simulink model "manual_model_features"  (R2020b)
settings: Solver=VariableStepAuto  StartTime=0.0  StopTime=10.0  RelTol=1e-3
undefined symbols (not defined in the file): sigbuilder_block
libraries: simulink x141
(part 3 of 3)

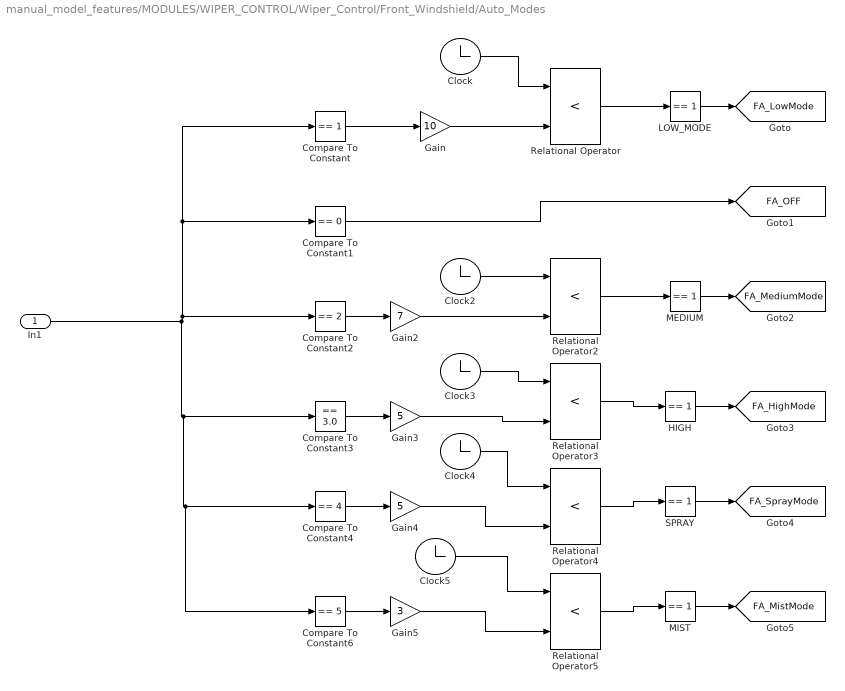
== system manual_model_features/MODULES/WIPER_CONTROL/Wiper_Control/Front_Windshield/Auto_Modes ==
  In1 : Inport
  Clock{,2..5} (5 alike) : Clock
      settings: Decimation=5
  Compare To Constant : simulink/Logic and Bit Operations/Compare To Constant  relop===  const=1  OutDataTypeStr=boolean
  Compare To Constant1 : simulink/Logic and Bit Operations/Compare To Constant  relop===  const=0  OutDataTypeStr=boolean
  Compare To Constant2 : simulink/Logic and Bit Operations/Compare To Constant  relop===  const=2  OutDataTypeStr=boolean
  Compare To Constant3 : simulink/Logic and Bit Operations/Compare To Constant  relop===  const=3.0  OutDataTypeStr=boolean
  Compare To Constant4 : simulink/Logic and Bit Operations/Compare To Constant  relop===  const=4  OutDataTypeStr=boolean
  Compare To Constant6 : simulink/Logic and Bit Operations/Compare To Constant  relop===  const=5  OutDataTypeStr=boolean
  Gain : Gain  Gain=10
  Gain2 : Gain  Gain=7
  Gain3 : Gain  Gain=5
  Gain4 : Gain  Gain=5
  Gain5 : Gain  Gain=3
  HIGH : simulink/Logic and Bit Operations/Compare To Constant  relop===  const=1  OutDataTypeStr=boolean
  LOW_MODE : simulink/Logic and Bit Operations/Compare To Constant  relop===  const=1  OutDataTypeStr=boolean
  MEDIUM : simulink/Logic and Bit Operations/Compare To Constant  relop===  const=1  OutDataTypeStr=boolean
  MIST : simulink/Logic and Bit Operations/Compare To Constant  relop===  const=1  OutDataTypeStr=boolean
  Relational Operator{,2..5} (5 alike) : RelationalOperator  Operator=<  OutDataTypeStr=boolean  RndMeth=Simplest
  SPRAY : simulink/Logic and Bit Operations/Compare To Constant  relop===  const=1  OutDataTypeStr=boolean
  tag scope: FA_HighMode=global, FA_LowMode=global, FA_MediumMode=global, FA_MistMode=global, FA_OFF=global, FA_SprayMode=global
  wires:
  In1/1 -> Compare To Constant6/1, Compare To Constant4/1, Compare To Constant3/1, Compare To Constant2/1, Compare To Constant/1, Compare To Constant1/1
  Clock/1 -> Relational Operator/1
  Relational Operator/1 -> LOW_MODE/1
  Gain/1 -> Relational Operator/2
  Compare To Constant/1 -> Gain/1
  Clock2/1 -> Relational Operator2/1
  Gain2/1 -> Relational Operator2/2
  Compare To Constant2/1 -> Gain2/1
  Clock3/1 -> Relational Operator3/1
  Gain3/1 -> Relational Operator3/2
  Compare To Constant3/1 -> Gain3/1
  Gain4/1 -> Relational Operator4/2
  Clock4/1 -> Relational Operator4/1
  Compare To Constant4/1 -> Gain4/1
  LOW_MODE/1 -> [FA_LowMode]
  MEDIUM/1 -> [FA_MediumMode]
  Relational Operator2/1 -> MEDIUM/1
  HIGH/1 -> [FA_HighMode]
  Relational Operator3/1 -> HIGH/1
  SPRAY/1 -> [FA_SprayMode]
  Relational Operator4/1 -> SPRAY/1
  Compare To Constant1/1 -> [FA_OFF]
  Relational Operator5/1 -> MIST/1
  Gain5/1 -> Relational Operator5/2
  Clock5/1 -> Relational Operator5/1
  MIST/1 -> [FA_MistMode]
  Compare To Constant6/1 -> Gain5/1

== system manual_model_features/MODULES/WIPER_CONTROL/Wiper_Control/Front_Windshield/Manual_mode ==
  In1 : Inport
  Bw30_60 : Logic  IconShape=distinctive  AllPortsSameDT=off  OutDataTypeStr=boolean
  Bw60_100 : Logic  IconShape=distinctive  AllPortsSameDT=off  OutDataTypeStr=boolean
  Compare To Constant1 : simulink/Logic and Bit Operations/Compare To Constant  relop=>  const=30  OutDataTypeStr=boolean
  Compare To Constant2 : simulink/Logic and Bit Operations/Compare To Constant  relop=<=  const=60  OutDataTypeStr=boolean
  Compare To Constant3 : simulink/Logic and Bit Operations/Compare To Constant  relop=>  const=60  OutDataTypeStr=boolean
  Compare To Constant4 : simulink/Logic and Bit Operations/Compare To Constant  relop=<=  const=100  OutDataTypeStr=boolean
  Display : Display
  LessThan30 : simulink/Logic and Bit Operations/Compare To Constant  relop=<=  const=30  OutDataTypeStr=boolean
  Slider : SliderBlock
  String Constant : StringConstant  String="\"Undefined!\""
  Switch : Switch  Criteria=u2 > Threshold  Threshold=5
  tag scope: FM_Bw30_60=global, FM_Bw60_100=global, FM_lessthan30=global
  wires:
  Compare To Constant1/1 -> Bw30_60/1
  Bw30_60/1 -> [FM_Bw30_60]
  [FC_ManualInput] -> Compare To Constant4/1, Compare To Constant3/1, Compare To Constant2/1, Compare To Constant1/1, LessThan30/1, Switch/1
  Compare To Constant4/1 -> Bw60_100/2
  LessThan30/1 -> [FM_lessthan30]
  Switch/1 -> Display/1
  Compare To Constant3/1 -> Bw60_100/1
  Bw60_100/1 -> [FM_Bw60_100]
  Compare To Constant2/1 -> Bw30_60/2
  In1/1 -> Switch/2
  String Constant/1 -> Switch/3

== system manual_model_features/MODULES/SeatRestraintSystem1/PowerLumbar/PowerSeat/Subsystem/RearAdjustmentLogic ==
  ConditionCheck : Inport
  Enable : EnablePort
  Adjusted : simulink/Logic and Bit Operations/Compare To Constant  relop=>  const=0  OutDataTypeStr=boolean
  Forward/RearSlide : Constant  Value=47.22916666666666
  Switch : Switch  Criteria=u2 > Threshold
  "adjustment : Front / Back1" : Display
  wires:
  ConditionCheck/1 -> Switch/2
  Forward/RearSlide/1 -> Switch/1
  Switch/1 -> Adjusted/1
  Adjusted/1 -> "adjustment : Front / Back1"/1

== system manual_model_features/MODULES/SeatRestraintSystem1/PowerLumbar/PowerSeat/Subsystem1/SeatAdjustmentLogic ==
  ConditionCheck : Inport
  Enable : EnablePort
  Compare To Constant : simulink/Logic and Bit Operations/Compare To Constant  relop=>  const=0  OutDataTypeStr=boolean
  SeatAdjust : Constant  Value=40.98647388059701
  Switch : Switch  Criteria=u2 > Threshold
  "adjustment : High/Low" : Display
  wires:
  ConditionCheck/1 -> Switch/2
  SeatAdjust/1 -> Switch/1
  Switch/1 -> Compare To Constant/1
  Compare To Constant/1 -> "adjustment : High/Low"/1

== system manual_model_features/MODULES/SeatRestraintSystem1/PowerLumbar/PowerSeat/Subsystem2/CushionAdjustmentLogic ==
  ConditionCheck : Inport
  Enable : EnablePort
  Compare To Constant : simulink/Logic and Bit Operations/Compare To Constant  relop=>  const=0  OutDataTypeStr=boolean
  CushionAdjust : Constant  Value=17.10587686567164
  Switch : Switch  Criteria=u2 > Threshold
  "adjustment : Cushion " : Display
  wires:
  ConditionCheck/1 -> Switch/2
  CushionAdjust/1 -> Switch/1
  Switch/1 -> Compare To Constant/1
  Compare To Constant/1 -> "adjustment : Cushion "/1

== stateflow chart manual_model_features/MODULES/	POWER_WINDOW/Subsystem4/Front_left_subsystem/decision_Box ==
  state Normal
    state Start
      entry:
      op1 = 25;
    state second
      entry:
      op1 = 100;
    state PrepareToStop
      entry:
      op1 = 75;
    state Go
      % Green light
      entry:
      op1 = 50;
    (default) -> Start
    Start -> (junction 9)
    (junction 9) -> (junction 6) : after(1,sec)
    PrepareToStop -> second : after(1,sec)
    (junction 6) -> Go
    Go -> PrepareToStop : after(1,sec)
  state Fault
    entry:
    op1 =0;
    state BlinkOn
      % Red light
      entry:
      warning = 1;
    (default) -> BlinkOn
  state block_start
    entry:
  state Normal2
    state state5
      entry:
      op1=0
    state Start1
      entry:
      op1=op1;
    state two
      entry:
      op1 = 0;
    state four3
      entry:
      op1 = 0;
    state three
      entry:
      op1 = 25;
    state three1
      entry:
      op1 = 0;
    state five2
      entry:
      op1=0;
    state five
      entry:
      op1=50;
    state five1
      entry:
      op1=25;
    state four2
      entry:
      op1 = 25;
    state four
      entry:
      op1 = 75;
    state four1
      entry:
      op1 = 50;
    Start1 -> state5 [order 4] : [op1==0]
    (default) -> Start1
    Start1 -> (junction 143) [order 2] : after(1,sec)[op1==25]
    (junction 143) -> four3
    Start1 -> (junction 89) [order 3]
    Start1 -> (junction 103) [order 5]
    Start1 -> (junction 48) [order 1]
    (junction 103) -> (junction 104) : after(1,sec)[op1==50]
    (junction 48) -> (junction 49) : after(1,sec)[op1==100]
    (junction 89) -> (junction 90) : after(1,sec)[op1==75]
    three -> two : after(1,sec)[op1==25]
    (junction 104) -> four2
    (junction 49) -> four
    five -> three : after(1,sec)[op1==50]
    (junction 90) -> four1
    five1 -> three1 : after(1,sec)[op1==25]
    four2 -> five2 : after(1,sec)[op1==25]
    four -> five : after(1,sec)[op1==75]
    four1 -> five1 : after(1,sec)[op1==50]
  (default) -> block_start
  block_start -> Normal2 [order 2] : [data == 0]
  Normal -> Fault [order 1] : [data1 == 1]
  block_start -> Normal [order 1] : [data ==1 ]
  Normal2 -> block_start [order 1] : [data ==1]
  Normal -> block_start [order 2] : [data == 0]
  Fault -> Normal [order 1] : [data1 == 0]
  Fault -> Normal2 [order 2] : [data1 ==0]
  Normal2 -> Fault [order 2] : [data1==1]
  data: data input; data1 input; op1 output =0; warning output

== stateflow chart manual_model_features/MODULES/	POWER_WINDOW/Subsystem4/Rear_right_Subsystem/Chart ==
  state Normal
    state Start
      entry:
      op1 = 25;
    state second
      entry:
      op1 = 100;
    state PrepareToStop
      entry:
      op1 = 75;
    state Go
      % Green light
      entry:
      op1 = 50;
    (default) -> Start
    Start -> (junction 9)
    (junction 9) -> (junction 6) : after(1,sec)
    PrepareToStop -> second : after(1,sec)
    (junction 6) -> Go
    Go -> PrepareToStop : after(1,sec)
  state Fault
    entry:
    op1 =0;
    state BlinkOn
      % Red light
      entry:
      warning = 1;
    (default) -> BlinkOn
  state block_start
    entry:
  state Normal2
    state state5
      entry:
      op1=0
    state Start1
      entry:
    state two
      entry:
      op1 = 0;
    state four3
      entry:
      op1 = 0;
    state three
      entry:
      op1 = 25;
    state three1
      entry:
      op1 = 0;
    state five2
      entry:
      op1=0;
    state five
      entry:
      op1=50;
    state five1
      entry:
      op1=25;
    state four2
      entry:
      op1 = 25;
    state four
      entry:
      op1 = 75;
    state four1
      entry:
      op1 = 50;
    Start1 -> state5 [order 2] : [op1==0]
    (default) -> Start1
    Start1 -> (junction 143) [order 3] : after(1,sec)[op1==25]
    (junction 143) -> four3
    Start1 -> (junction 89) [order 4]
    Start1 -> (junction 103) [order 5]
    Start1 -> (junction 48) [order 1]
    (junction 103) -> (junction 104) : after(1,sec)[op1==50]
    (junction 48) -> (junction 49) : after(1,sec)[op1==100]
    (junction 89) -> (junction 90) : after(1,sec)[op1==75]
    three -> two : after(1,sec)[op1==25]
    (junction 104) -> four2
    (junction 49) -> four
    five -> three : after(1,sec)[op1==50]
    (junction 90) -> four1
    five1 -> three1 : after(1,sec)[op1==25]
    four2 -> five2 : after(1,sec)[op1==25]
    four -> five : after(1,sec)[op1==75]
    four1 -> five1 : after(1,sec)[op1==50]
  (default) -> block_start
  block_start -> Normal2 [order 2] : [data == 0]
  Normal -> Fault [order 1] : [data1 == 1]
  block_start -> Normal [order 1] : [data ==1]
  Normal2 -> block_start [order 1] : [data ==1]
  Normal -> block_start [order 2] : [data ==0]
  Fault -> Normal [order 1] : [data1 == 0]
  Fault -> Normal2 [order 2] : [data1 ==0]
  Normal2 -> Fault [order 2] : [data1==1]
  data: data input; data1 input; op1 output =0; warning output

== stateflow chart manual_model_features/MODULES/Subsystem2/enabling system/Chart ==
  state stage1
    entry:
    enableO=0;
    enableC=0;
  state stage3
    entry:
    enableO=1;
    enableC=0;
  state stage2
    entry:
    enableO=0;
    enableC=1;
  (default) -> stage1
  stage1 -> stage3 [order 3] : [openButton ==1 && closeButton==0]
  stage1 -> stage2 [order 1] : [openButton ==0 && closeButton==1]
  stage2 -> stage1 : [(openButton ==1 && closeButton==1) || (openButton ==0 && closeButton==0)]
  stage3 -> stage1 : [(openButton ==1 && closeButton==1) || (openButton ==0 && closeButton==0)]
  stage1 -> stage1 [order 2] : [(openButton ==1 && closeButton==1) || (openButton ==0 && closeButton==0)]
  data: closeButton input; openButton input; enableC output; enableO output

== stateflow chart manual_model_features/MODULES/	POWER_WINDOW/Subsystem4/driver_control_Subsystem/Chart ==
  state Normal
    state Start
      entry:
      op1 = 25;
    state second
      entry:
      op1 = 100;
    state PrepareToStop
      entry:
      op1 = 75;
    state Go
      % Green light
      entry:
      op1 = 50;
    (default) -> Start
    Start -> (junction 9)
    (junction 9) -> (junction 6) : after(1,sec)
    PrepareToStop -> second : after(1,sec)
    (junction 6) -> Go
    Go -> PrepareToStop : after(1,sec)
  state Fault
    entry:
    op1 =0;
    state BlinkOn
      % Red light
      entry:
      warning = 1;
    (default) -> BlinkOn
  state block_start
    entry:
  state Normal2
    state state5
      entry:
      op1=0
    state Start1
      entry:
      op1=op1;
    state two
      entry:
      op1 = 0;
    state four3
      entry:
      op1 = 0;
    state three
      entry:
      op1 = 25;
    state three1
      entry:
      op1 = 0;
    state five2
      entry:
      op1=0;
    state five
      entry:
      op1=50;
    state five1
      entry:
      op1=25;
    state four2
      entry:
      op1 = 25;
    state four
      entry:
      op1 = 75;
    state four1
      entry:
      op1 = 50;
    Start1 -> state5 [order 4] : [op1==0]
    (default) -> Start1
    Start1 -> (junction 142) [order 2] : after(1,sec)[op1==25]
    Start1 -> (junction 89) [order 3]
    Start1 -> (junction 103) [order 5]
    (junction 142) -> four3
    Start1 -> (junction 48) [order 1]
    (junction 103) -> (junction 104) : after(1,sec)[op1==50]
    (junction 48) -> (junction 49) : after(1,sec)[op1==100]
    (junction 89) -> (junction 90) : after(1,sec)[op1==75]
    three -> two : after(1,sec)[op1==25]
    (junction 104) -> four2
    (junction 49) -> four
    five -> three : after(1,sec)[op1==50]
    (junction 90) -> four1
    five1 -> three1 : after(1,sec)[op1==25]
    four2 -> five2 : after(1,sec)[op1==25]
    four -> five : after(1,sec)[op1==75]
    four1 -> five1 : after(1,sec)[op1==50]
  (default) -> block_start
  block_start -> Normal2 [order 2] : [data == 0]
  Normal -> Fault [order 1] : [data1 == 1]
  block_start -> Normal [order 1] : [data ==1]
  Normal2 -> block_start [order 1] : [data ==1]
  Normal -> block_start [order 2] : [data ==0]
  Fault -> Normal [order 1] : [data1 == 0]
  Fault -> Normal2 [order 2] : [data1 ==0]
  Normal2 -> Fault [order 2] : [data1==1]
  data: data input; data1 input; op1 output =0; warning output

== stateflow chart manual_model_features/MODULES/	POWER_WINDOW/Subsystem4/rear_left_Subsystem/Chart ==
  state Normal
    state Start
      entry:
      op1 = 25;
    state second
      entry:
      op1 = 100;
    state PrepareToStop
      entry:
      op1 = 75;
    state Go
      % Green light
      entry:
      op1 = 50;
    (default) -> Start
    Start -> (junction 9)
    (junction 9) -> (junction 6) : after(1,sec)
    PrepareToStop -> second : after(1,sec)
    (junction 6) -> Go
    Go -> PrepareToStop : after(1,sec)
  state Fault
    entry:
    op1 =0;
    state BlinkOn
      % Red light
      entry:
      warning = 1;
    (default) -> BlinkOn
  state block_start
    entry:
  state Normal2
    state state5
      entry:
      op1=0
    state Start1
      entry:
      op1=op1;
    state two
      entry:
      op1 = 0;
    state four3
      entry:
      op1 = 0;
    state three
      entry:
      op1 = 25;
    state three1
      entry:
      op1 = 0;
    state five2
      entry:
      op1=0;
    state five
      entry:
      op1=50;
    state five1
      entry:
      op1=25;
    state four2
      entry:
      op1 = 25;
    state four
      entry:
      op1 = 75;
    state four1
      entry:
      op1 = 50;
    Start1 -> state5 [order 4] : [op1==0]
    (default) -> Start1
    Start1 -> (junction 142) [order 2] : after(1,sec)[op1==25]
    (junction 142) -> four3
    Start1 -> (junction 89) [order 3]
    Start1 -> (junction 103) [order 5]
    Start1 -> (junction 48) [order 1]
    (junction 103) -> (junction 104) : after(1,sec)[op1==50]
    (junction 48) -> (junction 49) : after(1,sec)[op1==100]
    (junction 89) -> (junction 90) : after(1,sec)[op1==75]
    three -> two : after(1,sec)[op1==25]
    (junction 104) -> four2
    (junction 49) -> four
    five -> three : after(1,sec)[op1==50]
    (junction 90) -> four1
    five1 -> three1 : after(1,sec)[op1==25]
    four2 -> five2 : after(1,sec)[op1==25]
    four -> five : after(1,sec)[op1==75]
    four1 -> five1 : after(1,sec)[op1==50]
  (default) -> block_start
  block_start -> Normal2 [order 2] : [data == 0]
  Normal -> Fault [order 1] : [data1 == 1]
  block_start -> Normal [order 1] : [data ==1]
  Normal2 -> block_start [order 1] : [data ==1]
  Normal -> block_start [order 2] : [data ==0]
  Fault -> Normal [order 1] : [data1 == 0]
  Fault -> Normal2 [order 2] : [data1 ==0]
  Normal2 -> Fault [order 2] : [data1==1]
  data: data input; data1 input; op1 output =0; warning output

== matlab function manual_model_features/MODULES/CRUISE_CONTROL/MATLAB Function ==
  data: ESC_CC input; TSC_CC input; BRAKE_CC input; IGN input; y output; DESIRED_SPEED_CRUISE input; cs input; CRUISE_SPEED_CHANGE_SW input; speedch input
function y = fcn(ESC_CC, TSC_CC, BRAKE_CC, IGN, DESIRED_SPEED_CRUISE, cs, CRUISE_SPEED_CHANGE_SW, speedch)

if (IGN==1&& ESC_CC==0 &&TSC_CC==0 && BRAKE_CC==0)
    if (cs ==1 && DESIRED_SPEED_CRUISE>40 && CRUISE_SPEED_CHANGE_SW==1)
        y= DESIRED_SPEED_CRUISE+speedch;
    else
        y=DESIRED_SPEED_CRUISE;
    end
      
else
    y=0;
end

== matlab function manual_model_features/MODULES/AirBagSystem/ActivateAirBagSensor ==
  data: SuddenDeceleration input; AirBagSensor output
function AirBagSensor  = fcn(SuddenDeceleration)
if SuddenDeceleration == 1
         %Front airbag active
   AirBagSensor = 1;
else 
   AirBagSensor = 0;   
end

== matlab function manual_model_features/MODULES/AirBagSystem/FrontAirBagActivation/WeightSensor ==
  data: driver input; DRIVER output; l_front input; L_FRONT output; l_rear input; r_rear input; L_REAR output; R_REAR output
function [DRIVER,L_FRONT,L_REAR,R_REAR] = fcn(driver, l_front,l_rear,r_rear)
    if (driver==0 && l_front==0 && l_rear==0 && r_rear==1)      %0001
        DRIVER=0;
        L_FRONT=0;
        L_REAR=0;
        R_REAR=1;
    
    elseif (driver==0 && l_front==0 && l_rear==1 && r_rear==0)
        DRIVER=0;
        L_FRONT=0;
        L_REAR=1;
        R_REAR=0;
    
    elseif (driver==0 && l_front==0 && l_rear==1 && r_rear==1)
        DRIVER=0;
        L_FRONT=0;
        L_REAR=1;
        R_REAR=1;

    elseif (driver==0 && l_front==1 && l_rear==0 && r_rear==0)
        DRIVER=0;
        L_FRONT=1;
        L_REAR=0;
        R_REAR=0;
    
    elseif (driver==0 && l_front==1 && l_rear==0 && r_rear==1)
        DRIVER=0;
        L_FRONT=1;
        L_REAR=0;
        R_REAR=1;
    
    elseif (driver==0 && l_front==1 && l_rear==1 && r_rear==0)
        DRIVER=0;
        L_FRONT=1;
        L_REAR=1;
        R_REAR=0;
    
    elseif (driver==0 && l_front==1 && l_rear==1 && r_rear==1)
        DRIVER=0;
        L_FRONT=1;
        L_REAR=1;
        R_REAR=1;
    
    elseif (driver==1 && l_front==0 && l_rear==0 && r_rear==0)
        DRIVER=1;
        L_FRONT=0;
        L_REAR=0;
        R_REAR=0;
    
    elseif (driver==1 && l_front==0 && l_rear==0 && r_rear==1)
        DRIVER=1;
        L_FRONT=0;
        L_REAR=0;
        R_REAR=1;
    
    elseif (driver==1 && l_front==0 && l_rear==1 && r_rear==0)
        DRIVER=1;
        L_FRONT=0;
        L_REAR=1;
        R_REAR=0;
    
    elseif (driver==1 && l_front==0 && l_rear==1 && r_rear==1)
        DRIVER=1;
        L_FRONT=0;
        L_REAR=1;
        R_REAR=1;
    
    elseif (driver==1 && l_front==1 && l_rear==0 && r_rear==0)
        DRIVER=1;
        L_FRONT=1;
        L_REAR=0;
        R_REAR=0;
    
    elseif (driver==1 && l_front==1 && l_rear==0 && r_rear==1)
        DRIVER=1;
        L_FRONT=1;
        L_REAR=0;
        R_REAR=1;
    
    elseif (driver==1 && l_front==1 && l_rear==1 && r_rear==0)
        DRIVER=1;
        L_FRONT=1;
        L_REAR=1;
        R_REAR=0;
    
    elseif (driver==1 && l_front==1 && l_rear==1 && r_rear==1)
        DRIVER=1;
        L_FRONT=1;
        L_REAR=1;
        R_REAR=1;
    
    else
        DRIVER=0;
        L_FRONT=0;
        L_REAR=0;
        R_REAR=0;
    end

== matlab function manual_model_features/MODULES/AirBagSystem/SideAirBagActivation/WeightSensor ==
  data: driver input; DRIVER output; l_front input; L_FRONT output; l_rear input; r_rear input; L_REAR output; R_REAR output
function [DRIVER,L_FRONT,L_REAR,R_REAR] = fcn(driver, l_front,l_rear,r_rear)
    if (driver==0 && l_front==0 && l_rear==0 && r_rear==1)      %0001
        DRIVER=0;
        L_FRONT=0;
        L_REAR=0;
        R_REAR=1;
    
    elseif (driver==0 && l_front==0 && l_rear==1 && r_rear==0)
        DRIVER=0;
        L_FRONT=0;
        L_REAR=1;
        R_REAR=0;
    
    elseif (driver==0 && l_front==0 && l_rear==1 && r_rear==1)
        DRIVER=0;
        L_FRONT=0;
        L_REAR=1;
        R_REAR=1;

    elseif (driver==0 && l_front==1 && l_rear==0 && r_rear==0)
        DRIVER=0;
        L_FRONT=1;
        L_REAR=0;
        R_REAR=0;
    
    elseif (driver==0 && l_front==1 && l_rear==0 && r_rear==1)
        DRIVER=0;
        L_FRONT=1;
        L_REAR=0;
        R_REAR=1;
    
    elseif (driver==0 && l_front==1 && l_rear==1 && r_rear==0)
        DRIVER=0;
        L_FRONT=1;
        L_REAR=1;
        R_REAR=0;
    
    elseif (driver==0 && l_front==1 && l_rear==1 && r_rear==1)
        DRIVER=0;
        L_FRONT=1;
        L_REAR=1;
        R_REAR=1;
    
    elseif (driver==1 && l_front==0 && l_rear==0 && r_rear==0)
        DRIVER=1;
        L_FRONT=0;
        L_REAR=0;
        R_REAR=0;
    
    elseif (driver==1 && l_front==0 && l_rear==0 && r_rear==1)
        DRIVER=1;
        L_FRONT=0;
        L_REAR=0;
        R_REAR=1;
    
    elseif (driver==1 && l_front==0 && l_rear==1 && r_rear==0)
        DRIVER=1;
        L_FRONT=0;
        L_REAR=1;
        R_REAR=0;
    
    elseif (driver==1 && l_front==0 && l_rear==1 && r_rear==1)
        DRIVER=1;
        L_FRONT=0;
        L_REAR=1;
        R_REAR=1;
    
    elseif (driver==1 && l_front==1 && l_rear==0 && r_rear==0)
        DRIVER=1;
        L_FRONT=1;
        L_REAR=0;
        R_REAR=0;
    
    elseif (driver==1 && l_front==1 && l_rear==0 && r_rear==1)
        DRIVER=1;
        L_FRONT=1;
        L_REAR=0;
        R_REAR=1;
    
    elseif (driver==1 && l_front==1 && l_rear==1 && r_rear==0)
        DRIVER=1;
        L_FRONT=1;
        L_REAR=1;
        R_REAR=0;
    
    elseif (driver==1 && l_front==1 && l_rear==1 && r_rear==1)
        DRIVER=1;
        L_FRONT=1;
        L_REAR=1;
        R_REAR=1;
    
    else
        DRIVER=0;
        L_FRONT=0;
        L_REAR=0;
        R_REAR=0;
    end

== stateflow chart manual_model_features/MODULES/ALARM_SYSTEM/ARMED ==
  state data
  state DELAY_1
    entry:
    data1 = 1;
  state DELAY
    entry:
    count=0;
    count = count + 1;
    data1 = 1;
  data -> DELAY_1 [order 2] : [data==1]
  (default) -> data
  data -> DELAY [order 1] : [data==0]
  DELAY -> DELAY : [count~=30]
  data: data input; data1 output; count local

== stateflow chart manual_model_features/MODULES/ALARM_SYSTEM/Main_Alarm/ARMED ==
  state data
  state DELAY_1
    entry:
    data1 = 1;
  state DELAY
    entry:
    count=0;
    count = count + 1;
    data1 = 1;
  data -> DELAY_1 [order 2] : [data==1]
  (default) -> data
  data -> DELAY [order 1] : [data==0]
  DELAY -> DELAY : [count~=30]
  data: data input; data1 output; count local

== stateflow chart manual_model_features/MODULES/ALARM_SYSTEM/Main_Alarm/Pre_Alarm ==
  state RKE1
    entry:
  state DELAY_3
    entry:
    data1 = 1;
  state DELAY_2
    entry:
    counter=0;
    counter = counter +1;
    data1 = 0;
  (default) -> RKE1
  RKE1 -> DELAY_3 [order 2] : [data==1]
  RKE1 -> DELAY_2 [order 1] : [data==0]
  DELAY_2 -> DELAY_2 : [counter~=10]
  data: data input; data1 output; counter local

== stateflow chart manual_model_features/MODULES/ALARM_SYSTEM/Pre_Alarm ==
  state RKE1
    entry:
  state DELAY_3
    entry:
    data1 = 1;
  state DELAY_2
    entry:
    counter=0;
    counter = counter +1;
    data1 = 0;
  (default) -> RKE1
  RKE1 -> DELAY_3 [order 2] : [data==1]
  RKE1 -> DELAY_2 [order 1] : [data==0]
  DELAY_2 -> DELAY_2 : [counter~=10]
  data: data input; data1 output; counter local

== matlab function manual_model_features/MODULES/AirBagSystem2/ActivateAirBagSensor ==
  data: SuddenDeceleration input; AirBagSensor output
function AirBagSensor  = fcn(SuddenDeceleration)
if SuddenDeceleration == 1
         %Front airbag active
   AirBagSensor = 1;
else 
   AirBagSensor = 0;   
end

== matlab function manual_model_features/MODULES/AirBagSystem2/FrontAirBagActivation/WeightSensor ==
  data: driver input; DRIVER output; l_front input; L_FRONT output; l_rear input; r_rear input; L_REAR output; R_REAR output
function [DRIVER,L_FRONT,L_REAR,R_REAR] = fcn(driver, l_front,l_rear,r_rear)
    if (driver==0 && l_front==0 && l_rear==0 && r_rear==1)      %0001
        DRIVER=0;
        L_FRONT=0;
        L_REAR=0;
        R_REAR=1;
    
    elseif (driver==0 && l_front==0 && l_rear==1 && r_rear==0)
        DRIVER=0;
        L_FRONT=0;
        L_REAR=1;
        R_REAR=0;
    
    elseif (driver==0 && l_front==0 && l_rear==1 && r_rear==1)
        DRIVER=0;
        L_FRONT=0;
        L_REAR=1;
        R_REAR=1;

    elseif (driver==0 && l_front==1 && l_rear==0 && r_rear==0)
        DRIVER=0;
        L_FRONT=1;
        L_REAR=0;
        R_REAR=0;
    
    elseif (driver==0 && l_front==1 && l_rear==0 && r_rear==1)
        DRIVER=0;
        L_FRONT=1;
        L_REAR=0;
        R_REAR=1;
    
    elseif (driver==0 && l_front==1 && l_rear==1 && r_rear==0)
        DRIVER=0;
        L_FRONT=1;
        L_REAR=1;
        R_REAR=0;
    
    elseif (driver==0 && l_front==1 && l_rear==1 && r_rear==1)
        DRIVER=0;
        L_FRONT=1;
        L_REAR=1;
        R_REAR=1;
    
    elseif (driver==1 && l_front==0 && l_rear==0 && r_rear==0)
        DRIVER=1;
        L_FRONT=0;
        L_REAR=0;
        R_REAR=0;
    
    elseif (driver==1 && l_front==0 && l_rear==0 && r_rear==1)
        DRIVER=1;
        L_FRONT=0;
        L_REAR=0;
        R_REAR=1;
    
    elseif (driver==1 && l_front==0 && l_rear==1 && r_rear==0)
        DRIVER=1;
        L_FRONT=0;
        L_REAR=1;
        R_REAR=0;
    
    elseif (driver==1 && l_front==0 && l_rear==1 && r_rear==1)
        DRIVER=1;
        L_FRONT=0;
        L_REAR=1;
        R_REAR=1;
    
    elseif (driver==1 && l_front==1 && l_rear==0 && r_rear==0)
        DRIVER=1;
        L_FRONT=1;
        L_REAR=0;
        R_REAR=0;
    
    elseif (driver==1 && l_front==1 && l_rear==0 && r_rear==1)
        DRIVER=1;
        L_FRONT=1;
        L_REAR=0;
        R_REAR=1;
    
    elseif (driver==1 && l_front==1 && l_rear==1 && r_rear==0)
        DRIVER=1;
        L_FRONT=1;
        L_REAR=1;
        R_REAR=0;
    
    elseif (driver==1 && l_front==1 && l_rear==1 && r_rear==1)
        DRIVER=1;
        L_FRONT=1;
        L_REAR=1;
        R_REAR=1;
    
    else
        DRIVER=0;
        L_FRONT=0;
        L_REAR=0;
        R_REAR=0;
    end

== matlab function manual_model_features/MODULES/AirBagSystem2/FrontAirBagActivation1/WeightSensor ==
  data: driver input; DRIVER output; l_front input; L_FRONT output; l_rear input; r_rear input; L_REAR output; R_REAR output
function [DRIVER,L_FRONT,L_REAR,R_REAR] = fcn(driver, l_front,l_rear,r_rear)
    if (driver==0 && l_front==0 && l_rear==0 && r_rear==1)      %0001
        DRIVER=0;
        L_FRONT=0;
        L_REAR=0;
        R_REAR=1;
    
    elseif (driver==0 && l_front==0 && l_rear==1 && r_rear==0)
        DRIVER=0;
        L_FRONT=0;
        L_REAR=1;
        R_REAR=0;
    
    elseif (driver==0 && l_front==0 && l_rear==1 && r_rear==1)
        DRIVER=0;
        L_FRONT=0;
        L_REAR=1;
        R_REAR=1;

    elseif (driver==0 && l_front==1 && l_rear==0 && r_rear==0)
        DRIVER=0;
        L_FRONT=1;
        L_REAR=0;
        R_REAR=0;
    
    elseif (driver==0 && l_front==1 && l_rear==0 && r_rear==1)
        DRIVER=0;
        L_FRONT=1;
        L_REAR=0;
        R_REAR=1;
    
    elseif (driver==0 && l_front==1 && l_rear==1 && r_rear==0)
        DRIVER=0;
        L_FRONT=1;
        L_REAR=1;
        R_REAR=0;
    
    elseif (driver==0 && l_front==1 && l_rear==1 && r_rear==1)
        DRIVER=0;
        L_FRONT=1;
        L_REAR=1;
        R_REAR=1;
    
    elseif (driver==1 && l_front==0 && l_rear==0 && r_rear==0)
        DRIVER=1;
        L_FRONT=0;
        L_REAR=0;
        R_REAR=0;
    
    elseif (driver==1 && l_front==0 && l_rear==0 && r_rear==1)
        DRIVER=1;
        L_FRONT=0;
        L_REAR=0;
        R_REAR=1;
    
    elseif (driver==1 && l_front==0 && l_rear==1 && r_rear==0)
        DRIVER=1;
        L_FRONT=0;
        L_REAR=1;
        R_REAR=0;
    
    elseif (driver==1 && l_front==0 && l_rear==1 && r_rear==1)
        DRIVER=1;
        L_FRONT=0;
        L_REAR=1;
        R_REAR=1;
    
    elseif (driver==1 && l_front==1 && l_rear==0 && r_rear==0)
        DRIVER=1;
        L_FRONT=1;
        L_REAR=0;
        R_REAR=0;
    
    elseif (driver==1 && l_front==1 && l_rear==0 && r_rear==1)
        DRIVER=1;
        L_FRONT=1;
        L_REAR=0;
        R_REAR=1;
    
    elseif (driver==1 && l_front==1 && l_rear==1 && r_rear==0)
        DRIVER=1;
        L_FRONT=1;
        L_REAR=1;
        R_REAR=0;
    
    elseif (driver==1 && l_front==1 && l_rear==1 && r_rear==1)
        DRIVER=1;
        L_FRONT=1;
        L_REAR=1;
        R_REAR=1;
    
    else
        DRIVER=0;
        L_FRONT=0;
        L_REAR=0;
        R_REAR=0;
    end
